simulink model "VDC25_old"  (R2022a)
settings: Solver=FixedStepAuto  StartTime=0.0  StopTime=10.0  FixedStep=vdc_TimeStep  RelTol=1e-3
undefined symbols (not defined in the file): DiscIntNeverNeededParam, pac, param, param_vdc, vx0, vy0, yaw_rate0
settings Model: Creator=jutri  LastModifiedBy=Usuario
settings ModelReferenceCC: EnableRefExpFcnMdlSchedulingChecks=off
settings RTWCC: Description=Generic Real-Time Target  GPUComputeCapability=5.0

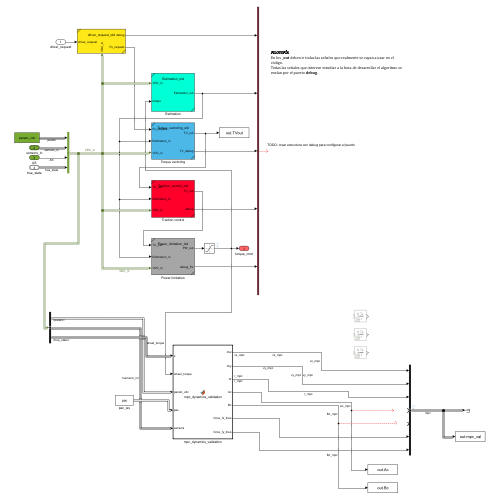
[thumbnail: Simulink's stored preview of the top-level diagram]
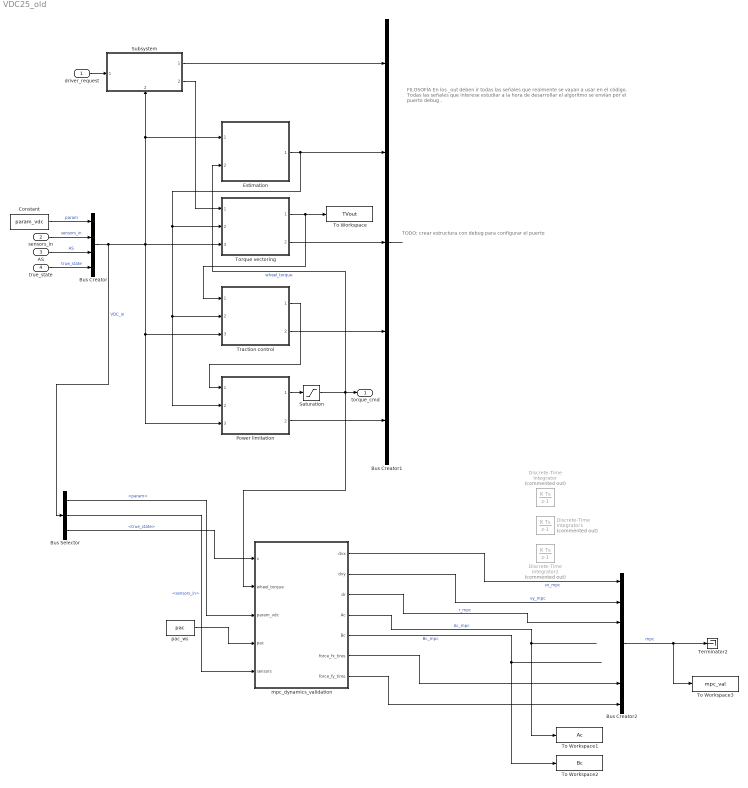
== system VDC25_old ==
  note: TODO: crear estructura con debug para configurar el puerto
  note: FILOSOFÍA
      | En los _out deben ir todas las señales que realmente se vayan a usar en el código.
      | Todas las señales que interese estudiar a la hora de desarrollar el algoritmo se envían por el puerto debug .
  driver_request : Inport
  sensors_in : Inport  Port=2  OutDataTypeStr=Bus: sensorBus
  AS : Inport  Port=3
  true_state : Inport  Port=4  OutDataTypeStr=Bus: stateBus
  Bus Creator : BusCreator  Inputs=4
  Bus Creator1 : BusCreator  Inputs=5
  Bus Creator2 : BusCreator  Inputs=7
  Bus Selector : BusSelector  OutputSignals=param,sensors_in,true_state
  Constant : Constant  Value=param_vdc  OutDataTypeStr=Bus: vdcBus
  Discrete-Time Integrator : DiscreteIntegrator  Commented=on  InitialCondition=vx0  SampleTime=-1  ICPrevOutput=DiscIntNeverNeededParam  ICPrevScaledInput=DiscIntNeverNeededParam
  Discrete-Time Integrator1 : DiscreteIntegrator  Commented=on  InitialCondition=vy0  SampleTime=-1  ICPrevOutput=DiscIntNeverNeededParam  ICPrevScaledInput=DiscIntNeverNeededParam
  Discrete-Time Integrator2 : DiscreteIntegrator  Commented=on  InitialCondition=yaw_rate0  SampleTime=-1  ICPrevOutput=DiscIntNeverNeededParam  ICPrevScaledInput=DiscIntNeverNeededParam
  Estimation : Subsystem  ReferencedSubsystem=Estimation_old
  Power limitation : Subsystem  ReferencedSubsystem=Power_limitation_old
  Saturation : Saturate  UpperLimit=param.torque_limit_positive  LowerLimit=param.torque_limit_negative
  Subsystem : Subsystem  ReferencedSubsystem=driver_request_old
      settings: PortSchema="{\"entries\":[{\"content\":{\"sides\":[{\"content\":{\"connectorIds\":[\"In1\"]},\"type\":\"ConnectorPlacement.EquallySpacedRectSide\",\"uuid\":\"6d0b78b3-ffc0-496d-8d3a-7ba3f556f803\"},{\"content\":{\"connectorIds\":[\"Out1\",\"Out2\"],\"side\":\"RIGHT\"},\"type\":\"ConnectorPlacement.EquallySpacedRectSide\",\"uuid\":\"be1dfba9-3592-437e-9363-a3609142bbc4\"},{\"content\":{\"connectorIds\":[],\"side\":\"TOP\"},\"type\":\"ConnectorPlacement.EquallySpacedRectSide\",\"uuid\":\"ddffd853-c46f-4213-b654-9451d95e6853\"},{\"content\":{\"connectorIds\":[\"In2\"],\"side\":\"BOTTOM\"},\"type\":\"ConnectorPlacement.EquallySpacedRectSide\",\"uuid\":\"b463dc20-ae30-4837-a1c3-1d0c4501f548\"}]},\"type\":\"ConnectorPlacement.EquallySpacedConnector\",\"uuid\":\"75a8dd9f-93ed-4a7a-b725-fd6938405663\"}],\"packageUris\":[\"http://schema.mathworks.com/mf0/Connector/R2020b\"],\"version\":\"1.0\"}"
  Terminator2 : Terminator
  To Workspace : ToWorkspace  VariableName=TVout  SaveFormat=Structure With Time  SampleTime=-1
  To Workspace1 : ToWorkspace  VariableName=Ac  SaveFormat=Structure With Time  SampleTime=-1
  To Workspace2 : ToWorkspace  VariableName=Bc  SaveFormat=Structure With Time  SampleTime=-1
  To Workspace3 : ToWorkspace  VariableName=mpc_val  SaveFormat=Structure With Time  SampleTime=-1
  Torque vectoring : Subsystem  ReferencedSubsystem=Torque_vectoring_old
  Traction control : Subsystem  ReferencedSubsystem=Traction_control_old
  mpc_dynamics_validation : MATLAB Function  TreatAsAtomicUnit=on
  pac_ws : Constant  Value=pac  OutDataTypeStr=Bus: pacBus
  torque_cmd : Outport
  wires:
  driver_request/1 -> Subsystem/1
  Bus Creator/1 -> Bus Selector/1, Power limitation/3, Traction control/3, Subsystem/2, Estimation/1, Torque vectoring/3  "VDC_in"
  Constant/1 -> Bus Creator/1  "param"
  sensors_in/1 -> Bus Creator/2  "sensors_in"
  AS/1 -> Bus Creator/3  "AS"
  Torque vectoring/1 -> To Workspace/1, Traction control/1
  Traction control/1 -> Power limitation/1
  Subsystem/2 -> Torque vectoring/1
  Subsystem/1 -> Bus Creator1/1
  Estimation/1 -> Torque vectoring/2, Traction control/2, Power limitation/2, Bus Creator1/2
  Torque vectoring/2 -> Bus Creator1/3
  Traction control/2 -> Bus Creator1/4
  Power limitation/2 -> Bus Creator1/5
  Power limitation/1 -> Saturation/1
  true_state/1 -> Bus Creator/4  "true_state"
  Bus Creator1/1 -> ?
  pac_ws/1 -> mpc_dynamics_validation/4(pac)
  mpc_dynamics_validation/2(dvy) -> Bus Creator2/2  "vy_mpc"
  mpc_dynamics_validation/1(dvx) -> Bus Creator2/1  "vx_mpc"
  Bus Selector/3 -> mpc_dynamics_validation/1(x)  "<true_state>"
  Bus Creator2/1 -> To Workspace3/1, Terminator2/1  "mpc"
  Bus Selector/2 -> mpc_dynamics_validation/5(sensors)  "<sensors_in>"
  mpc_dynamics_validation/3(dr) -> Bus Creator2/3  "r_mpc"
  Saturation/1 -> torque_cmd/1, mpc_dynamics_validation/2(wheel_torque), Estimation/2  "wheel_torque"
  Bus Selector/1 -> mpc_dynamics_validation/3(param_vdc)  "<param>"
  mpc_dynamics_validation/4(Ac) -> To Workspace1/1  "Ac_mpc"
  mpc_dynamics_validation/5(Bc) -> To Workspace2/1  "Bc_mpc"
  mpc_dynamics_validation/6(force_fx_tires) -> Bus Creator2/6
  mpc_dynamics_validation/7(force_fy_tires) -> Bus Creator2/7

== matlab function VDC25_old/mpc_dynamics_validation ==
  data: x input; dvx output; wheel_torque input; param_vdc input; pac input; sensors input; dvy output; dr output; Ac output; Bc output; force_fx_tires output; force_fy_tires output
function [dvx,dvy,dr,Ac,Bc, force_fx_tires, force_fy_tires] = mpc_dynamics_validation(x, wheel_torque, param_vdc, pac, sensors)

% Definimos valores instantáneos de las variables
vx = x.vx;
vy = x.vy;
yaw_rate = x.r;

% Definimos el estado actual y la actuación actual
x_k = [vx; vy; yaw_rate];
u_k = wheel_torque;

% Tamaños del sistema reducido para el MPC
nx = 3;
nu = 4;

Ac = zeros(nx, nx);
Bc = zeros(nx, nu);
Ad = zeros(nx, nx);
Bd = zeros(nx, nu);

% Definimos el valor de los sensores y su matriz
wheel_speed = [sensors.encoder.wFL; sensors.encoder.wFR; sensors.encoder.wRL; sensors.encoder.wRR];
dvx = sensors.IMU.ax;
dvy = sensors.IMU.ay;
delta_cmd = sensors.ext.steering;
vx_fijo = sensors.gss.vx;
sensors_in = [wheel_speed; delta_cmd; dvx; dvy; vx_fijo];

% Paso de perturbación (un valor muy pequeño pero mayor a epsilon)
delta = 1e-5;

for j = 1:nx
    x_plus = x_k;
    x_plus(j) = x_plus(j) + delta;
    dx_plus = f_dynamics(x_plus, u_k, sensors_in, param_vdc, pac, 0); 
    x_minus = x_k;
    x_minus(j) = x_minus(j) - delta;
    dx_minus = f_dynamics(x_minus, u_k, sensors_in, param_vdc, pac, 0);
    Ac(:, j) = (dx_plus - dx_minus) / (2 * delta);
end
for j = 1:nu
    u_plus = u_k;
    u_plus(j) = u_plus(j) + delta;
    dx_plus = f_dynamics(x_k, u_plus, sensors_in, param_vdc, pac, 0);
    u_minus = u_k;
    u_minus(j) = u_minus(j) - delta;
    dx_minus = f_dynamics(x_k, u_minus, sensors_in, param_vdc, pac, 0);
    Bc(:, j) = (dx_plus - dx_minus) / (2 * delta);
end

u_k = wheel_torque;

% x_k = [sensors.gss.vx; sensors.gss.vy; sensors.gss.r];
x_k = [vx; vy; yaw_rate];

% M = expm([Ac, Bc; zeros(nu, nx+nu)] .* 0.0050);
% Ad = M(1:nx, 1:nx);
% Bd = M(1:nx, nx+1:end);

% En lugar de expm:
Ad = eye(nx) + Ac .* 0.0050;
Bd = Bc .* 0.0050;

% Predicción a un paso
% x_out = Ad * x_k + Bd * u_k;

dx_nolineal_actual = f_dynamics(x_k, u_k, sensors_in, param_vdc, pac, 0);

% Residuo de linealización (La "d" escondida)
% Este término compensa el hecho de que no linealizamos en (0,0)
residual = dx_nolineal_actual - (Ac * x_k + Bc * u_k);

% Integramos ese residuo discretamente
d_k = residual .* 0.0050;

% 3. Ecuación de predicción LTV-MPC (como en el paper, ajustando la base)
x_out = Ad * x_k + Bd * u_k + d_k;

% wheel_speed = [x.wFL; x.wFR; x.wRL; x.wRR];
% dvx = x.ax;
% dvy = x.ay;
% delta_cmd = sensors.ext.steering;
% sensors_in = [wheel_speed; delta_cmd; dvx; dvy];

% dx_real_k = f_dynamics(x_k, u_k, sensors_in, param_vdc, pac, 0);
% 
% x_out = x_k + dx_real_k * 0.005;

dvx = x_out(1);
dvy = x_out(2);
dr = x_out(3);

[~, force_fx_tires, force_fy_tires] = f_dynamics(x_k, u_k, sensors_in, param_vdc, pac, 0);

end
